simulink model "spacartest"  (R2020b)
settings: Solver=VariableStepAuto  StartTime=0.0  StopTime=1  RelTol=1e-3
undefined symbols (not defined in the file or in its folder): spacar_lib, SPASIM
settings Model: Creator=Rick  LastModifiedBy=Rick

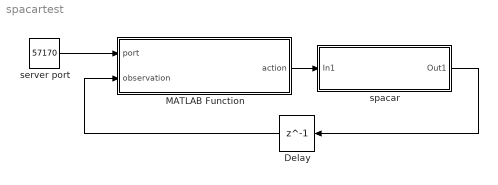
== system spacartest ==
  Delay : Delay  DelayLength=1  InitialCondition=[0; 0; 0; 0; 0; 0]
  MATLAB Function : MATLAB Function  TreatAsAtomicUnit=on
  server port : Constant  Value=57170
  spacar : Subsystem  AncestorBlock=spacar_lib/SPASIM  mask{filename='bicycle', use_spadraw=off, output_sbd=off}
      mask prompts: filename "SPACAR data filename"; use_spadraw "Visualize with spadraw"; output_sbd "Write SBD file"
      mask init:
      | if size(who('filenm'))>0; dfilenm=filenm; else; dfilenm=''; end
      mask Display: disp(filename);
  wires:
  server port/1 -> MATLAB Function/1(port)
  MATLAB Function/1(action) -> spacar/1(In1)
  Delay/1 -> MATLAB Function/2(observation)
  spacar/1(Out1) -> Delay/1

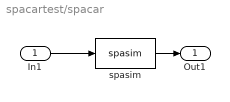
== system spacartest/spacar ==
  In1 : Inport  PortDimensions=3
  spasim : S-Function  FunctionName=spasim  Parameters=filename,use_spadraw,output_sbd  SFunctionDeploymentMode=off  EnableBusSupport=off
  Out1 : Outport  InitialOutput=0  VectorParamsAs1DForOutWhenUnconnected=off
  wires:
  spasim/1 -> Out1/1
  In1/1 -> spasim/1

== matlab function spacartest/MATLAB Function ==
  data: action output; port input; observation input
function action = tcp_comms(port, observation)
    coder.extrinsic('communicate');
    
    action = [0; 0; 0];
    action = communicate(port, observation);
end
